simulink model "KinematicBlocks"  (R2018b)
settings: Solver=ode4  StartTime=0.0  StopTime=10.0  FixedStep=0.001  RelTol=1e-3
settings Model: Creator=Asus  LastModifiedBy=batuhantoker

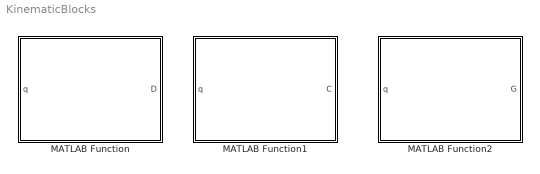
== system KinematicBlocks ==
  MATLAB Function : MATLAB Function  TreatAsAtomicUnit=on
  MATLAB Function1 : MATLAB Function  TreatAsAtomicUnit=on
  MATLAB Function2 : MATLAB Function  TreatAsAtomicUnit=on

== matlab function KinematicBlocks/MATLAB Function1 ==
  data: q input; C output
function C = Coriolis_Matrix(q)


I1 = [290212.21, 0, 0; 0, 275331.77, 0; 0, 0, 509323.35];
I2 = [7409.27 0 0; 0 52876.31 -0.01; 0 -0.01 50680.51];
I3 = [3801.21 -0.03 -0.24; -0.03 87085.96 -0.02; -0.24 -0.02 86685.11];
m1 = 258.22;
m2 = 57.56;
m3 = 47.17;

mA = m1;
mB = m2;
mC = m3;

IA11 = I1(1,1);
IA12 = I1(1,2);
IA13 = I1(1,3);
IA21 = I1(2,1);
IA22 = I1(2,2);
IA23 = I1(2,3);
IA31 = I1(3,1);
IA32 = I1(3,2);
IA33 = I1(3,3);

IB11 = I2(1,1);
IB12 = I2(1,2);
IB13 = I2(1,3);
IB21 = I2(2,1);
IB22 = I2(2,2);
IB23 = I2(2,3);
IB31 = I2(3,1);
IB32 = I2(3,2);
IB33 = I2(3,3);

IC11 = I3(1,1);
IC12 = I3(1,2);
IC13 = I3(1,3);
IC21 = I3(2,1);
IC22 = I3(2,2);
IC23 = I3(2,3);
IC31 = I3(3,1);
IC32 = I3(3,2);
IC33 = I3(3,3);

q1 = q(1);
q2 = q(2);
q3 = q(3);

c11 = cos(q2)*(IB31*cos(q2)-2437.6881917025*mB*sin(q2))+2*sin(q2+q3)*(IC11*cos(q2+q3)-IC31*sin(q2+q3))...
    +2*cos(q2+q3)*(IC31*cos(q2+q3)-IC33*sin(q2+q3))+sin(q2)*(IB11*cos(q2)-IB31*sin(q2)-IB33*cos(q2))...
    -6924.635234220001*mC*(sin(q3+ 2 * q2) + 1.408125112298184 * sin(q2) * cos(q2)) ...
    - 6924.635234220001 * mC * sin(q2 + q3) * (cos(q2) + 1.420328337682881 * cos(q2 + q3));

c12 = IB23 * sin(q2) + 2 * IC23 * sin(q2 + q3) + cos(q2) * (IB31 * cos(q2)... 
    - 2437.6881917025 * mB * sin(q2)) + sin(q2 + q3) * (IC11 * cos(q2 + q3) - IC31 * sin(q2 + q3)) ...
    + cos(q2 + q3) * (IC31 * cos(q2 + q3) - IC33 * sin(q2 + q3))...
    + sin(q2) * (IB11 * cos(q2) - IB31 * sin(q2) - IB33 * cos(q2)) ...
    - IB12 * cos(q2) - 2 * IC12 * cos(q2 + q3) ...
    - 4917.62782564 * mC * (1.408125112298184 * sin(q3 + 2 * q2) ...
    + 1.982816331884774 * sin(q2) * cos(q2) + sin(q2 + q3) * cos(q2 + q3));

c13 = 2 * IC23 * sin(q2 + q3) + sin(q2 + q3) * (IC11 * cos(q2 + q3) - IC31 * sin(q2 + q3)) ...
    + cos(q2 + q3) * (IC31 * cos(q2 + q3) - IC33 * sin(q2 + q3)) - 2 * IC12 * cos(q2 + q3) ...
    - 4917.62782564 * mC * sin(q2 + q3) * (cos(q2 + q3) + 1.408125112298184 * cos(q2));

c21 = 4917.62782564 * mC * (1.408125112298184 * sin(q3 + 2 * q2) ...
    + 1.982816331884774 * sin(q2) * cos(q2) + sin(q2 + q3) * cos(q2 + q3)) ...
    - cos(q2) * (IB31 * cos(q2) - 2437.6881917025 * mB * sin(q2)) ...
    - sin(q2 + q3) * (IC11 * cos(q2 + q3) - IC31 * sin(q2 + q3)) ...
    -cos(q2 + q3) * (IC31 * cos(q2 + q3) - IC33 * sin(q2 + q3)) ...
    - sin(q2) * (IB11 * cos(q2) - IB31 * sin(q2) - IB33 * cos(q2));

c22 = -6924.63523422 * mC * sin(q3);

c23 = -13849.27046844 * mC * sin(q3);

c31 = 4917.62782564 * mC * sin(q2 + q3) * (cos(q2 + q3) + 1.408125112298184 * cos(q2))...
    - sin(q2 + q3) * (IC11 * cos(q2 + q3) - IC31 * sin(q2 + q3)) ...
    - cos(q2 + q3) * (IC31 * cos(q2 + q3) - IC33 * sin(q2 + q3));

c32 = 6924.63523422 * mC * sin(q3);

c33 = 0;

C = [c11, c12, c13; c21, c22, c23; c31, c32, c33];

== matlab function KinematicBlocks/MATLAB Function ==
  data: q input; D output
function D = Inertia_Matrix(q)

I1 = [290212.21, 0, 0; 0, 275331.77, 0; 0, 0, 509323.35];
I2 = [7409.27 0 0; 0 52876.31 -0.01; 0 -0.01 50680.51];
I3 = [3801.21 -0.03 -0.24; -0.03 87085.96 -0.02; -0.24 -0.02 86685.11];

m1 = 258.22;
m2 = 57.56;
m3 = 47.17;

mA = m1;
mB = m2;
mC = m3;

IA11 = I1(1,1);
IA12 = I1(1,2);
IA13 = I1(1,3);
IA21 = I1(2,1);
IA22 = I1(2,2);
IA23 = I1(2,3);
IA31 = I1(3,1);
IA32 = I1(3,2);
IA33 = I1(3,3);

IB11 = I2(1,1);
IB12 = I2(1,2);
IB13 = I2(1,3);
IB21 = I2(2,1);
IB22 = I2(2,2);
IB23 = I2(2,3);
IB31 = I2(3,1);
IB32 = I2(3,2);
IB33 = I2(3,3);

IC11 = I3(1,1);
IC12 = I3(1,2);
IC13 = I3(1,3);
IC21 = I3(2,1);
IC22 = I3(2,2);
IC23 = I3(2,3);
IC31 = I3(3,1);
IC32 = I3(3,2);
IC33 = I3(3,3);

q1 = q(1);
q2 = q(2);
q3 = q(3);

m11 = IA33 + IB33 + IC33 + 2437.6881917025 * mB  ...
    + 4917.62782564 * mC * (cos(q2 + q3)^2 + 1.982816331884774 * cos(q2)^2 ...
    + 2.816250224596368 * cos(q2) * cos(q2 + q3)) + sin(q2 + q3) * (IC11 * sin(q2 + q3) ...
    + 2 * IC31 * cos(q2 + q3) - IC33 - sin(q2 + q3)) + sin(q2) - (IB11 - sin(q2) ...
    + 2 * IB31 * cos(q2) - 2437.6881917025 * mB * sin(q2) - IB33 * sin(q2));

m12 = -IB12 * sin(q2) - IB23 * cos(q2) - IC12 * sin(q2 + q3) - IC23 * cos(q2 + q3);
m13 = -IC12 * sin(q2 + q3) - IC23 * cos(q2 + q3);
m21 = -IB12 * sin(q2) - IB23 * cos(q2) - IC12 * sin(q2 + q3) - IC23 * cos(q2 + q3);
m22 = IB22 + IC22 + 2437.6881917025 * mB + 13849.27046844 * mC * (1.059144640569812 + cos(q3));
m23 = IC22 + 4917.62782564 * mC * (1 + 1.408125112298184 * cos(q3));
m31 = -IC12 * sin(q2 + q3) - IC23 * cos(q2 + q3);
m32 = IC22 + 4917.62782564 * mC * (1 + 1.408125112298184 * cos(q3));
m33 = IC22 + 4917.62782564 * mC;

D = [m11, m12, m13; m21, m22, m23; m31, m32, m33];

== matlab function KinematicBlocks/MATLAB Function2 ==
  data: q input; G output
function G = Gravity(q)
m1 = 258.22;
m2 = 57.56;
m3 = 47.17;

mA = m1;
mB = m2;
mC = m3;

q1 = q(1);
q2 = q(2);
q3 = q(3);


g = 9810;
g1 = 0;
g2 = 49.37295 * g * (mB + 2 * mC) * cos(q2);
g3 = 70.1258 * g * mC * cos(q3);

G = [g1; g2; g3];
